simulink model "routing"  (R2022a)
settings: Solver=VariableStepAuto  StartTime=0.0  StopTime=10.0  RelTol=1e-3
settings Model: Creator=vfton  LastModifiedBy=vfton

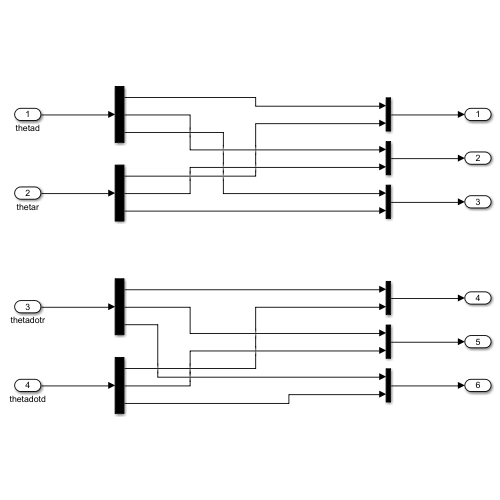
[thumbnail: Simulink's stored preview of the top-level diagram]
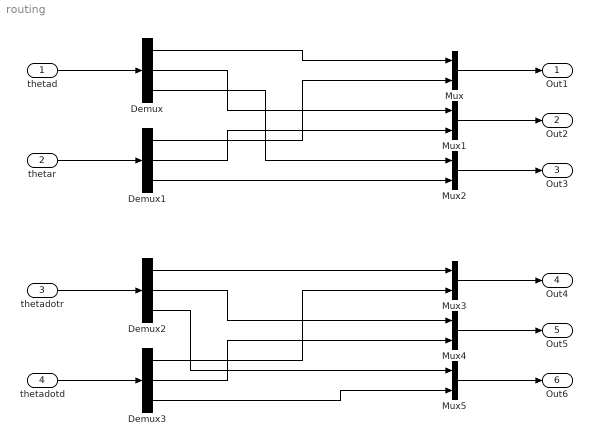
== system routing ==
  thetad : Inport
  thetar : Inport  Port=2
  thetadotr : Inport  Port=3
  thetadotd : Inport  Port=4
  Demux{,1..3} (4 alike) : Demux  Outputs=3
  Mux{,1..5} (6 alike) : Mux  Inputs=2
  Out1 : Outport
  Out2 : Outport  Port=2
  Out3 : Outport  Port=3
  Out4 : Outport  Port=4
  Out5 : Outport  Port=5
  Out6 : Outport  Port=6
  wires:
  thetad/1 -> Demux/1
  thetar/1 -> Demux1/1
  thetadotr/1 -> Demux2/1
  thetadotd/1 -> Demux3/1
  Demux/1 -> Mux/1
  Demux1/1 -> Mux/2
  Demux/2 -> Mux1/1
  Demux1/2 -> Mux1/2
  Demux/3 -> Mux2/1
  Demux1/3 -> Mux2/2
  Demux2/1 -> Mux3/1
  Demux3/1 -> Mux3/2
  Demux2/2 -> Mux4/1
  Demux3/2 -> Mux4/2
  Demux2/3 -> Mux5/1
  Demux3/3 -> Mux5/2
  Mux3/1 -> Out4/1
  Mux4/1 -> Out5/1
  Mux5/1 -> Out6/1
  Mux2/1 -> Out3/1
  Mux1/1 -> Out2/1
  Mux/1 -> Out1/1
